simulink subsystem "Navigation"  (R2021a)
settings: Solver=VariableStepAuto  StartTime=0.0  StopTime=10.0  RelTol=1e-3
settings Model: Creator=Laura  LastModifiedBy=Laura

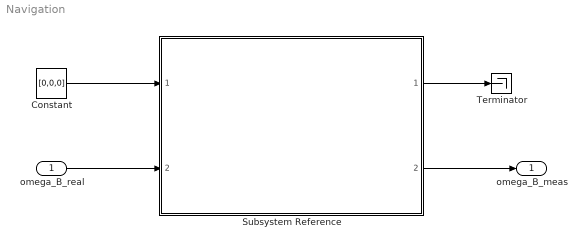
== system Navigation ==
  omega_B_real : Inport
  Constant : Constant  Value=[0,0,0]
  Subsystem Reference : Subsystem  ReferencedSubsystem=ADIS16460
  Terminator : Terminator
  omega_B_meas : Outport
  wires:
  Constant/1 -> Subsystem Reference/1
  omega_B_real/1 -> Subsystem Reference/2
  Subsystem Reference/2 -> omega_B_meas/1
  Subsystem Reference/1 -> Terminator/1
